simulink model "symulacja"  (R2017a)
settings: Solver=VariableStepAuto  StartTime=0.0  StopTime=10  MaxStep=0.01  RelTol=1e-3
undefined symbols (not defined in the file or in its folder): A0, A120, A150, A180, A30, A60, A90, B0, B120, B150, B180, B30, B60, B90, K0, K30, K60
libraries: fuzblock x3
settings Model: Creator=Szwank  LastModifiedBy=Szwank

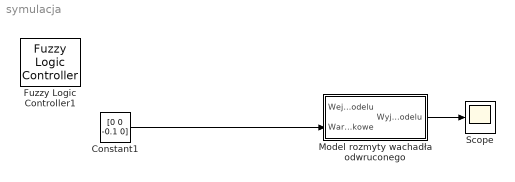
== system symulacja ==
  Constant1 : Constant  Value=[0 0 -0.1 0]
  Fuzzy Logic Controller1 : fuzblock/Fuzzy Logic  Controller  fis=['ProbaRegulator.fis']
  Model rozmyty wachadła odwruconego : Subsystem
  Scope : Scope
  wires:
  Constant1/1 -> Model rozmyty wachadła odwruconego/2(Warunki początkowe)
  Model rozmyty wachadła odwruconego/1(Wyjście Modelu) -> Scope/1

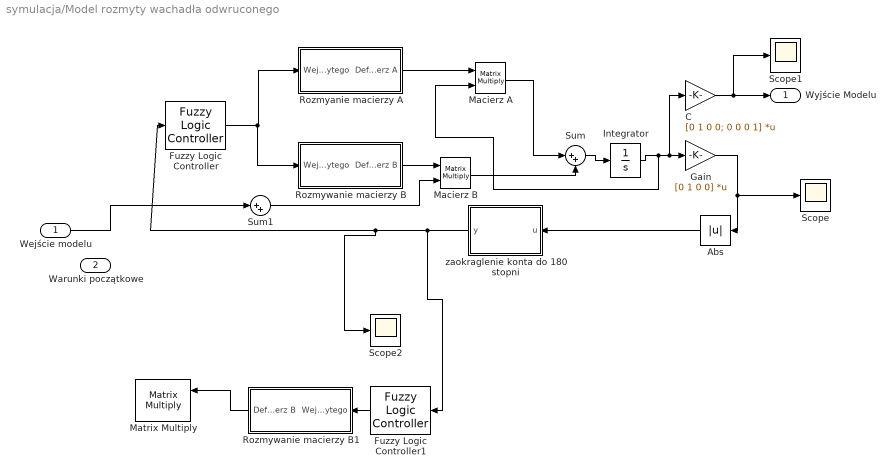
== system symulacja/Model rozmyty wachadła odwruconego ==
  Wejście modelu : Inport
  Warunki początkowe : Inport  Port=2
  Abs : Abs
  "C " : Gain  Gain=[0 1 0 0; 0 0 0 1]  Multiplication=Matrix(K*u)
  Fuzzy Logic Controller : fuzblock/Fuzzy Logic  Controller  fis=['modelRozmyty.fis']
  Fuzzy Logic Controller1 : fuzblock/Fuzzy Logic  Controller  fis=['modelRozmyty.fis']
  Gain : Gain  Gain=[0 1 0 0]  Multiplication=Matrix(K*u)
  Integrator : Integrator  InitialCondition=[0 0 1 0]
  Macierz A : Product  Multiplication=Matrix(*)
  Macierz B : Product  Multiplication=Matrix(*)
  Matrix Multiply : Product  Multiplication=Matrix(*)
  Rozmyanie macierzy A : Subsystem
  Rozmywanie macierzy B : Subsystem
  Rozmywanie macierzy B1 : Subsystem
  Scope : Scope
  Scope1 : Scope
  Scope2 : Scope
  Sum : Sum  Inputs=|++
  Sum1 : Sum  Inputs=|++
  "zaokraglenie konta do 180 stopni " : MATLAB Function  TreatAsAtomicUnit=on
  Wyjście Modelu : Outport
  wires:
  "C "/1 -> Scope1/1, Wyjście Modelu/1
  Rozmyanie macierzy A/1(Defuzyfikowana macierz A) -> Macierz A/1
  Gain/1 -> Scope/1, Abs/1
  Sum/1 -> Integrator/1
  Macierz A/1 -> Sum/1
  Macierz B/1 -> Sum/2
  Fuzzy Logic Controller/1 -> Rozmywanie macierzy B/1(Wejście z modelu rozmytego), Rozmyanie macierzy A/1(Wejście z modelu rozmytego)
  Abs/1 -> "zaokraglenie konta do 180 stopni "/1(u)
  Wejście modelu/1 -> Sum1/1
  Fuzzy Logic Controller1/1 -> Rozmywanie macierzy B1/1(Wejście z modelu rozmytego)
  Integrator/1 -> "C "/1, Gain/1, Macierz A/2
  "zaokraglenie konta do 180 stopni "/1(y) -> Fuzzy Logic Controller1/1, Scope2/1, Fuzzy Logic Controller/1
  Rozmywanie macierzy B1/1(Defuzyfikowana macierz B) -> Matrix Multiply/1
  Rozmywanie macierzy B/1(Defuzyfikowana macierz B) -> Macierz B/1
  Sum1/1 -> Macierz B/2

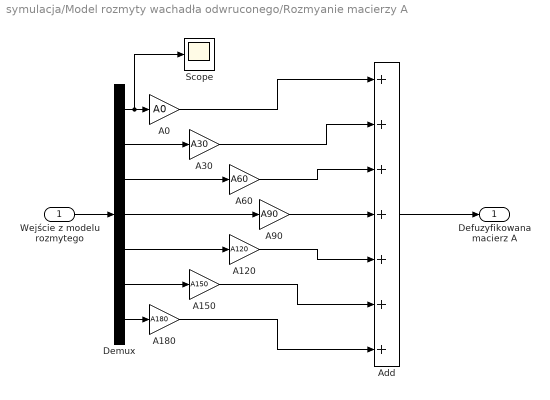
== system symulacja/Model rozmyty wachadła odwruconego/Rozmyanie macierzy A ==
  Wejście z modelu rozmytego : Inport
  A0 : Gain  Gain=A0
  A120 : Gain  Gain=A120
  A150 : Gain  Gain=A150
  A180 : Gain  Gain=A180
  A30 : Gain  Gain=A30
  A60 : Gain  Gain=A60
  A90 : Gain  Gain=A90
  Add : Sum  Inputs=+++++++
  Demux : Demux  Outputs=7
  Scope : Scope
  Defuzyfikowana macierz A : Outport
  wires:
  Demux/6 -> A150/1
  Demux/1 -> Scope/1, A0/1
  Wejście z modelu rozmytego/1 -> Demux/1
  Demux/2 -> A30/1
  Demux/7 -> A180/1
  Demux/5 -> A120/1
  Demux/4 -> A90/1
  Demux/3 -> A60/1
  A90/1 -> Add/4
  A0/1 -> Add/1
  A30/1 -> Add/2
  A60/1 -> Add/3
  A120/1 -> Add/5
  A150/1 -> Add/6
  A180/1 -> Add/7
  Add/1 -> Defuzyfikowana macierz A/1

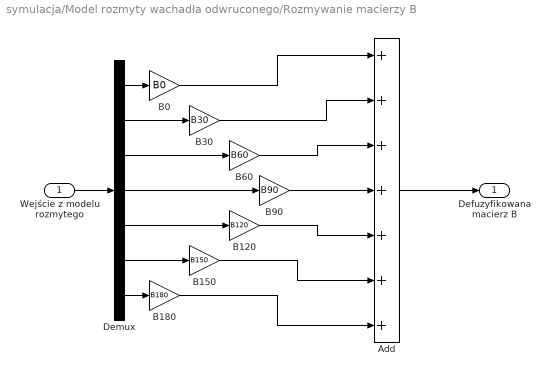
== system symulacja/Model rozmyty wachadła odwruconego/Rozmywanie macierzy B ==
  Wejście z modelu rozmytego : Inport
  Add : Sum  Inputs=+++++++
  B0 : Gain  Gain=B0
  B120 : Gain  Gain=B120
  B150 : Gain  Gain=B150
  B180 : Gain  Gain=B180
  B30 : Gain  Gain=B30
  B60 : Gain  Gain=B60
  B90 : Gain  Gain=B90
  Demux : Demux  Outputs=7
  Defuzyfikowana macierz B : Outport
  wires:
  Demux/6 -> B150/1
  Demux/1 -> B0/1
  Wejście z modelu rozmytego/1 -> Demux/1
  Demux/2 -> B30/1
  Demux/7 -> B180/1
  Demux/5 -> B120/1
  Demux/4 -> B90/1
  Demux/3 -> B60/1
  B90/1 -> Add/4
  B0/1 -> Add/1
  B30/1 -> Add/2
  B60/1 -> Add/3
  B120/1 -> Add/5
  B150/1 -> Add/6
  B180/1 -> Add/7
  Add/1 -> Defuzyfikowana macierz B/1

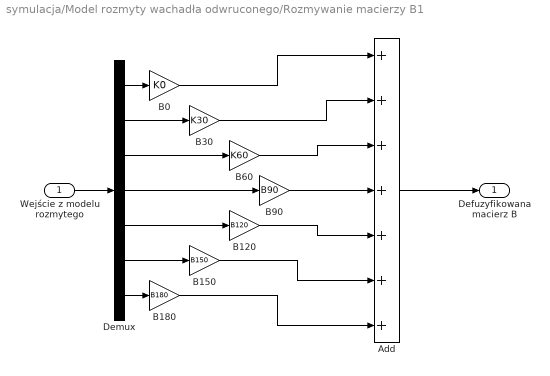
== system symulacja/Model rozmyty wachadła odwruconego/Rozmywanie macierzy B1 ==
  Wejście z modelu rozmytego : Inport
  Add : Sum  Inputs=+++++++
  B0 : Gain  Gain=K0
  B120 : Gain  Gain=B120
  B150 : Gain  Gain=B150
  B180 : Gain  Gain=B180
  B30 : Gain  Gain=K30
  B60 : Gain  Gain=K60
  B90 : Gain  Gain=B90
  Demux : Demux  Outputs=7
  Defuzyfikowana macierz B : Outport
  wires:
  Demux/6 -> B150/1
  Demux/1 -> B0/1
  Wejście z modelu rozmytego/1 -> Demux/1
  Demux/2 -> B30/1
  Demux/7 -> B180/1
  Demux/5 -> B120/1
  Demux/4 -> B90/1
  Demux/3 -> B60/1
  B90/1 -> Add/4
  B0/1 -> Add/1
  B30/1 -> Add/2
  B60/1 -> Add/3
  B120/1 -> Add/5
  B150/1 -> Add/6
  B180/1 -> Add/7
  Add/1 -> Defuzyfikowana macierz B/1

== matlab function symulacja/Model rozmyty wachadła odwruconego/zaokraglenie konta do 180 stopni  ==
  data: u input; y output
function y = fcn(u)

g = 180*u/pi;%zamiana na kat
if(g>180)
    reszta=rem(g,180);
    if(rem(fix(g/180),2)==1)
        g=180-reszta;
    else
        g=reszta;
    end
end

y = g;
